simulink model "HW2_1"  (R2021a)
settings: Solver=VariableStepAuto  StartTime=0.0  StopTime=4  RelTol=1e-3
settings Model: Creator=jhart  LastModifiedBy=jhart

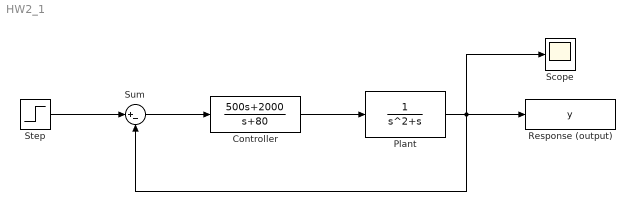
== system HW2_1 ==
  Controller : TransferFcn  Numerator=[500 2000]  Denominator=[1 80]
  Plant : TransferFcn  Denominator=[1 1 0]
  Response (output) : ToWorkspace  VariableName=y  SampleTime=-1
  Scope : Scope
  Step : Step  Time=0  SampleTime=0
  Sum : Sum  Inputs=|+-
  wires:
  Step/1 -> Sum/1
  Sum/1 -> Controller/1
  Controller/1 -> Plant/1
  Plant/1 -> Response (output)/1, Scope/1, Sum/2
